simulink model "fig3_23_simulink"  (R2021b)
settings: Solver=ode45  StartTime=0.0  StopTime=100  RelTol=1e-3  EnableMultiTasking=on
settings Model: Creator=One Informatic  LastModifiedBy=One Informatic
settings SolverCC: AlgebraicLoopSolver=TrustRegion
settings DataIOCC: LimitDataPoints=on  SaveFormat=Array  SignalLoggingSaveFormat=ModelDataLogs  ReturnWorkspaceOutputs=off
settings OptimizationCC: InitFltsAndDblsToZero=on  LifeSpan=inf
settings DebuggingCC: SaveWithParameterizedLinksMsg=none  UnderspecifiedInitializationDetection=Classic  MergeDetectMultiDrivingBlocksExec=none  SignalResolutionControl=TryResolveAllWithWarning  SolverPrmCheckMsg=warning  MultiTaskDSMMsg=warning  MultiTaskCondExecSysMsg=none  FcnCallInpInsideContextMsg=warning  SFUnexpectedBacktrackingDiag=warning  SFNoUnconditionalDefaultTransitionDiag=warning  SFExecutionAtInitializationDiag=none  SFMachineParentedDataDiag=warning  ArithmeticOperatorsInVariantConditions=warning
settings HardwareCC: ProdBitPerPointer=32  ProdBitPerSizeT=32  ProdBitPerPtrDiffT=32  ProdLargestAtomicFloat=None  ProdIntDivRoundTo=Undefined  ProdEndianess=Unspecified  ProdWordSize=32  ProdHWDeviceType=32-bit Generic
settings ModelReferenceCC: PropagateSignalLabelsOutOfModel=off
settings CodeAppCC: StateflowObjectComments=on
settings GRTTargetCC: TargetFcnLib=ansi_tfl_tmw.mat  TargetLangStandard=C89/C90 (ANSI)  CombineOutputUpdateFcns=off  GRTInterface=on
settings ConfigComp: CovMetricSettings=dw  CovSaveCumulativeToWorkspaceVar=on  CovSaveSingleToWorkspaceVar=on

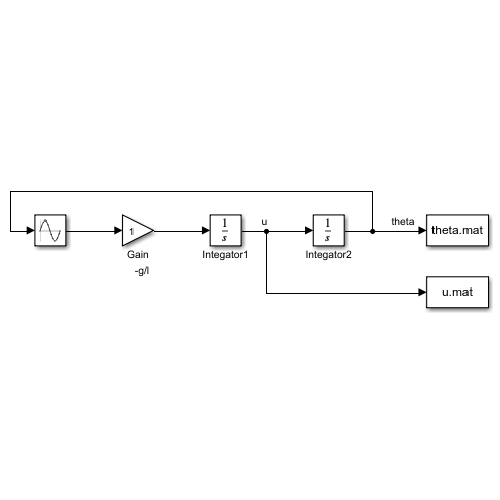
[thumbnail: Simulink's stored preview of the top-level diagram]
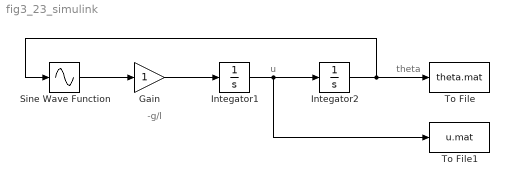
== system fig3_23_simulink ==
  note: u
  note: -g/l
  note: theta
  Gain : Gain
  Integator1 : Integrator  InitialCondition=0.2
  Integator2 : Integrator
  Sine Wave Function : Sin  TimeSource=Use external signal  SampleTime=0
  To File : ToFile  Filename=theta.mat  MatrixName=theta  SampleTime=0.001
  To File1 : ToFile  Filename=u.mat  MatrixName=u  SampleTime=0.001
  wires:
  Integator2/1 -> Sine Wave Function/1, To File/1
  Integator1/1 -> To File1/1, Integator2/1
  Sine Wave Function/1 -> Gain/1
  Gain/1 -> Integator1/1
